simulink model "cruise_control_sdo"  (Simulink 8.0)
settings: Solver=FixedStepDiscrete  SolverMode=SingleTasking  StartTime=0.0  StopTime=50  FixedStep=0.01  RelTol=1e-3  AbsTol=1e-6
model workspace (MAT data in the model file):
  converter_data = [0  137.465208994  2.232; 0.1  137.065019157  2.075; 0.2  135.864449646  1.975; 0.3  135.664354728  1.846; 0.4  137.565256453  1.72; 0.5  140.366585312  1.564; 0.6  145.268910814  1.409; 0.7  152.872517717  1.254; 0.8  162.9773111  1.096; 0.81  164.27792807  1.08; 0.82  166.178829795  1.061; 0.83  167.979684062  1.043; 0.84  170.080680706  1.028; 0.85  172.781962105  1.012; 0.86  175.383196045  1.002; 0.87  179.585189333  1.002; 0.88  183.587087703  1.001; 0.89  189.890077635  0.998; 0.9  197.693779455  0.999; 0.92  215.902417037  1.001; 0.94  244.515990379  1.002]
  emap = [-40  -44  -49  -53  -57  -61  -65  -70  -74  -78  -82; 215  117  85  66  44  29  10  -2  -13  -22  -32; 245  208  178  148  122  104  85  66  48  33  18; 264  260  241  219  193  167  152  133  119  96  85; 264  279  282  275  260  238  223  208  189  171  152; 267  290  293  297  290  275  260  256  234  212  193; 267  297  305  305  305  301  293  282  267  249  226; 267  301  308  312  319  323  319  316  297  279  253; 267  301  312  319  327  327  327  327  312  293  267; 267  301  312  319  327  334  334  334  319  305  275]
  Iei = 0.0219914882836
  nevec = [800 1200 1600 2000 2400 2800 3200 3600 4000 4400 4800]
  p0 = 0.07934
  p1 = 0.07934
  thvec = [0; 20; 30; 40; 50; 60; 70; 80; 90; 100]
  vehicledata : num (value not decoded)
values from neighbouring files (symbols this model uses):
  cruise_ki = 0.01    [cruise_control_data.m]    (also in fxpdata_simulinkpackage.mat)
  cruise_kp = 0.02    [cruise_control_data.m]    (also in fxpdata_simulinkpackage.mat)
  target_max = 100    [cruise_control_data.m]    (also in fxpdata_simulinkpackage.mat)
  target_min = 30    [cruise_control_data.m]    (also in fxpdata_simulinkpackage.mat)
  throt_max = 100    [cruise_control_data.m]    (also in fxpdata_simulinkpackage.mat)
  throt_min = 0    [cruise_control_data.m]    (also in fxpdata_simulinkpackage.mat)
  vel_dec = 1    [cruise_control_data.m]    (also in fxpdata_simulinkpackage.mat)
  vel_inc = 1    [cruise_control_data.m]    (also in fxpdata_simulinkpackage.mat)
libraries: simulink x1
Description:
  | 幚憰梡僋儖?[僘僐儞僩???[儖儌僨儖
settings Model: MinMaxOverflowLogging=MinMaxAndOverflow  Creator=The MathWorks Inc.  LastModifiedBy=hualongy  CovMetricSettings=dcmtr  CovHTMLOptions=-aTS=1 -bRG=1 -bTC=1 -hTR=0 -nFC=0 -scm=1 -bcm=1 -xEv=0  ExtModeTrigMode=oneshot  ExtModeArmWhenConnect=off  ExtModeAutoUpdateStatusClock=off
settings DataIOCC: LimitDataPoints=off  SignalLoggingSaveFormat=ModelDataLogs  SaveOutput=off  SaveTime=off  SignalLoggingName=mysig
settings OptimizationCC: InlineParams=on  UseIntDivNetSlope=on  UseSpecifiedMinMax=on  InlineInvariantSignals=on  EnhancedBackFolding=on  PassReuseOutputArgsAs=Individual arguments  ZeroExternalMemoryAtStartup=off  ZeroInternalMemoryAtStartup=off  NoFixptDivByZeroProtection=on  EfficientFloat2IntCast=on  OptimizeModelRefInitCode=on  LifeSpan=1
settings DebuggingCC: SignalInfNanChecking=error  SaveWithParameterizedLinksMsg=none  CheckExecutionContextPreStartOutputMsg=on  CheckExecutionContextRuntimeOutputMsg=on  SolverPrmCheckMsg=none  SingleTaskRateTransMsg=error  IntegerOverflowMsg=error  FcnCallInpInsideContextMsg=EnableAllAsWarning  UniqueDataStoreMsg=error  BusObjectLabelMismatch=error  RootOutportRequireBusObject=error  AssertControl=DisableAll  StrictBusMsg=ErrorOnBusTreatedAsVector  BusNameAdapt=ErrorWithoutRepair  NonBusSignalsTreatedAsBus=error  LoggingUnavailableSignals=none
settings HardwareCC: ProdIntDivRoundTo=Zero  ProdEndianess=LittleEndian  ProdHWDeviceType=NEC->V850  TargetIntDivRoundTo=Zero  TargetEndianess=LittleEndian  TargetHWDeviceType=MATLAB Host
settings ModelReferenceCC: ModelReferenceNumInstancesAllowed=Single
settings SFSimCC: SFSimEcho=off  SimParseCustomCode=off
settings RTWCC: SystemTargetFile=ert.tlc  TemplateMakefile=ert_default_tmf  Description=Embedded Coder  GenerateReport=on  ProcessScript=ert_make_rtw_hook  IncludeHyperlinkInReport=on  LaunchReport=on  GenerateErtSFunction=on  CreateSILPILBlock=SIL  IncludeERTFirstTime=on  GenerateTraceInfo=on  GenerateTraceReport=on  GenerateTraceReportSl=on  GenerateTraceReportSf=on  GenerateTraceReportEml=on  RTWCompilerOptimization=On
settings CodeAppCC: IgnoreCustomStorageClasses=off  IgnoreTestpoints=on
settings ERTTargetCC: CodeReplacementLibrary=ANSI_C  UtilityFuncGeneration=Shared location  MultiwordLength=2048  GenerateSampleERTMain=on  IncludeMdlTerminateFcn=off  CombineSignalStateStructs=on  SuppressErrorStatus=on  SupportNonFinite=off  SupportComplex=off  PurelyIntegerCode=on  ParenthesesLevel=Maximum  InlinedParameterPlacement=NonHierarchical  ERTCustomFileTemplate=example_file_process.tlc  SuppressUnreachableDefaultCases=off
settings ConfigComp: Description=Design Verifier Custom Configuration Component  DVMaxProcessTime=3000  DVDisplayUnsatisfiableObjectives=on  DVMakeOutputFilesUnique=off  DVModelCoverageObjectives=MCDC  DVMaxTestCaseSteps=500  DVTestSuiteOptimization=CombinedObjectives (Nonlinear Extended)  DVSaveExpectedOutput=on  DVSaveHarnessModel=on  DVModelReferenceHarness=on  DVSaveReport=on

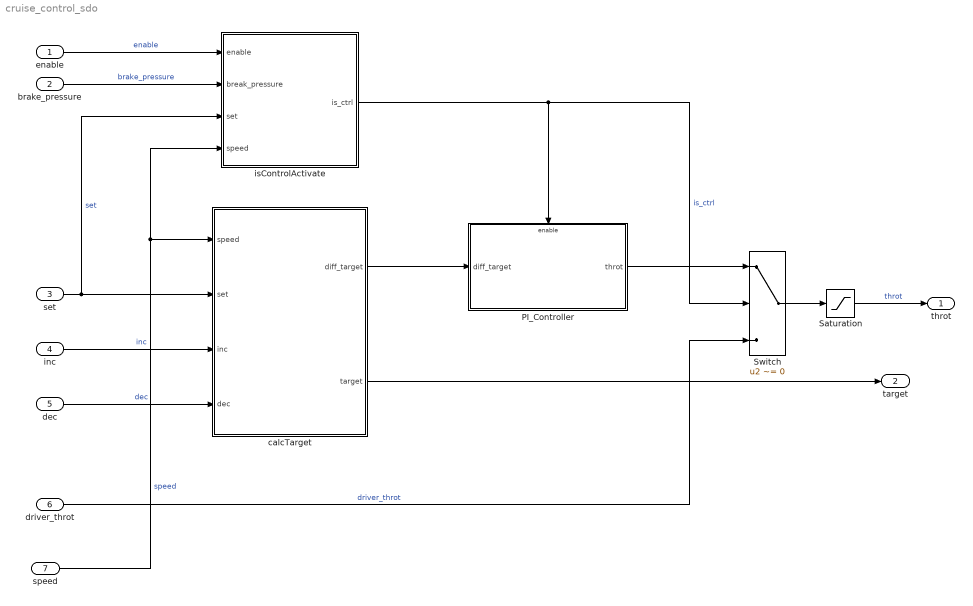
== system cruise_control_sdo ==
  enable : Inport  PortDimensions=1  Interpolate=off
  brake_pressure : Inport  Port=2  PortDimensions=1  Interpolate=off
  set : Inport  Port=3  PortDimensions=1  Interpolate=off
  inc : Inport  Port=4  PortDimensions=1  Interpolate=off
  dec : Inport  Port=5  PortDimensions=1  Interpolate=off
  driver_throt : Inport  Port=6  PortDimensions=1  Interpolate=off
  speed : Inport  Port=7  PortDimensions=1  Interpolate=off
  PI_Controller : Subsystem
  Saturation : Saturate  UpperLimit=throt_max  LowerLimit=throt_min  LinearizeAsGain=off  OutDataTypeStr=Inherit: Inherit via back propagation  RndMeth=Simplest
      settings: AttributesFormatString=<UpperLimit = %<UpperLimit>>\n<LowerLimit = %<LowerLimit>>
  Switch : Switch  Criteria=u2 ~= 0  OutDataTypeStr=Inherit: Inherit via back propagation
      settings: AttributesFormatString=<Criteria=%<Criteria>>
  calcTarget : Subsystem
  isControlActivate : Subsystem
  throt : Outport  PortDimensions=[1 1]
  target : Outport  Port=2  PortDimensions=[1 1]
  wires:
  isControlActivate/1(is_ctrl) -> Switch/2, PI_Controller/Enable  "is_ctrl"
  calcTarget/2(target) -> target/1
  calcTarget/1(diff_target) -> PI_Controller/1(diff_target)
  dec/1 -> calcTarget/4(dec)  "dec"
  speed/1 -> isControlActivate/4(speed), calcTarget/1(speed)  "speed"
  inc/1 -> calcTarget/3(inc)  "inc"
  set/1 -> isControlActivate/3(set), calcTarget/2(set)  "set"
  Switch/1 -> Saturation/1
  driver_throt/1 -> Switch/3  "driver_throt"
  brake_pressure/1 -> isControlActivate/2(break_pressure)  "brake_pressure"
  enable/1 -> isControlActivate/1(enable)  "enable"
  PI_Controller/1(throt) -> Switch/1
  Saturation/1 -> throt/1  "throt"

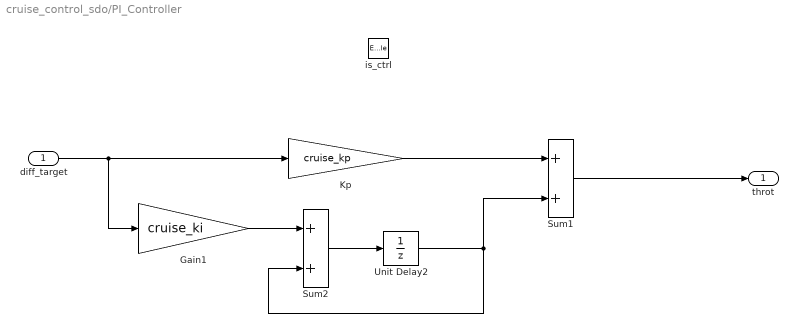
== system cruise_control_sdo/PI_Controller ==
  diff_target : Inport
  is_ctrl : EnablePort  StatesWhenEnabling=reset
  Gain1 : Gain  Gain=cruise_ki  OutDataTypeStr=Inherit: Same as input
  Kp : Gain  Gain=cruise_kp  ParamDataTypeStr=Inherit: Inherit from 'Gain'  OutDataTypeStr=Inherit: Inherit via back propagation
  Sum1 : Sum  OutDataTypeStr=Inherit: Inherit via back propagation
  Sum2 : Sum  OutDataTypeStr=Inherit: Inherit via back propagation
  Unit Delay2 : UnitDelay  SampleTime=-1
  throt : Outport
  wires:
  Unit Delay2/1 -> Sum2/2, Sum1/2
  Gain1/1 -> Sum2/1
  Kp/1 -> Sum1/1
  Sum1/1 -> throt/1
  diff_target/1 -> Gain1/1, Kp/1
  Sum2/1 -> Unit Delay2/1

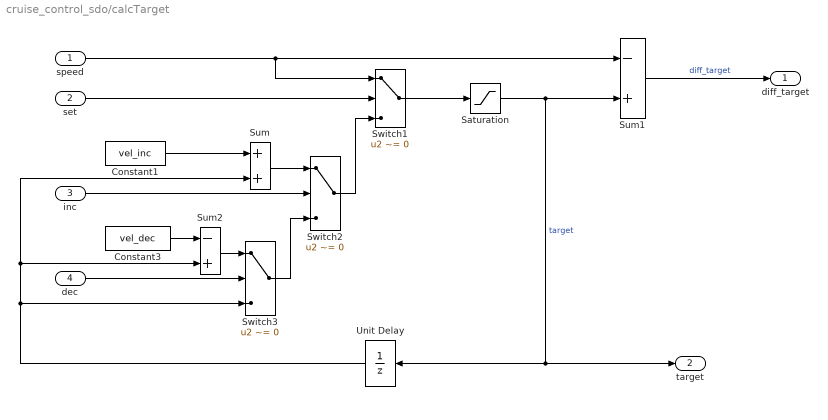
== system cruise_control_sdo/calcTarget ==
  speed : Inport
  set : Inport  Port=2
  inc : Inport  Port=3
  dec : Inport  Port=4
  Constant1 : Constant  Value=vel_inc  OutDataTypeStr=Inherit: Inherit via back propagation
  Constant3 : Constant  Value=vel_dec  OutDataTypeStr=Inherit: Inherit via back propagation
  Saturation : Saturate  UpperLimit=target_max  LowerLimit=target_min  LinearizeAsGain=off  RndMeth=Simplest
      settings: AttributesFormatString=<UpperLimit = %<UpperLimit>>\n<LowerLimit = %<LowerLimit>>
  Sum : Sum
  Sum1 : Sum  Inputs=-+  OutDataTypeStr=Inherit: Same as first input
  Sum2 : Sum  Inputs=-+
  Switch1 : Switch  Criteria=u2 ~= 0
      settings: AttributesFormatString=<Criteria=%<Criteria>>
  Switch2 : Switch  Criteria=u2 ~= 0
      settings: AttributesFormatString=<Criteria=%<Criteria>>
  Switch3 : Switch  Criteria=u2 ~= 0
      settings: AttributesFormatString=<Criteria=%<Criteria>>
  Unit Delay : UnitDelay  SampleTime=-1
  diff_target : Outport
  target : Outport  Port=2
  wires:
  Saturation/1 -> Sum1/2, target/1, Unit Delay/1  "target"
  set/1 -> Switch1/2
  speed/1 -> Switch1/1, Sum1/1
  inc/1 -> Switch2/2
  Constant1/1 -> Sum/1
  Sum/1 -> Switch2/1
  dec/1 -> Switch3/2
  Constant3/1 -> Sum2/1
  Sum2/1 -> Switch3/1
  Switch2/1 -> Switch1/3
  Switch3/1 -> Switch2/3
  Unit Delay/1 -> Switch3/3, Sum2/2, Sum/2
  Switch1/1 -> Saturation/1
  Sum1/1 -> diff_target/1  "diff_target"

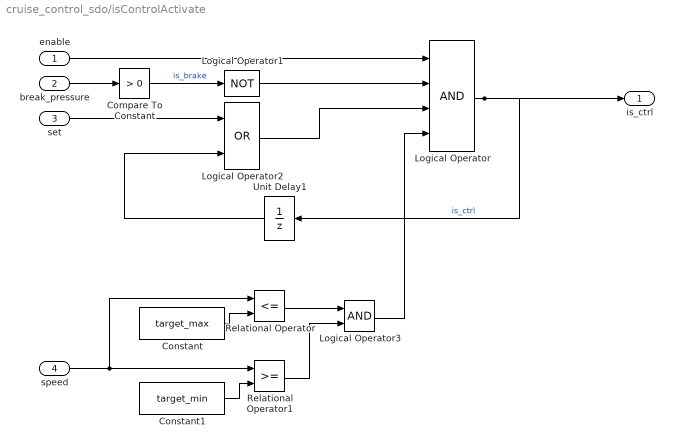
== system cruise_control_sdo/isControlActivate ==
  enable : Inport
  break_pressure : Inport  Port=2
  set : Inport  Port=3
  speed : Inport  Port=4
  Compare To Constant : simulink/Logic and Bit Operations/Compare To Constant  relop=>  const=0  OutDataTypeStr=uint8
  Constant : Constant  Value=target_max
  Constant1 : Constant  Value=target_min
  Logical Operator : Logic  Inputs=4  AllPortsSameDT=off  OutDataTypeStr=boolean
  Logical Operator1 : Logic  Operator=NOT  AllPortsSameDT=off  OutDataTypeStr=boolean
  Logical Operator2 : Logic  Operator=OR  AllPortsSameDT=off  OutDataTypeStr=boolean
  Logical Operator3 : Logic  AllPortsSameDT=off  OutDataTypeStr=boolean
  Relational Operator : RelationalOperator  Operator=<=  OutDataTypeStr=boolean
  Relational Operator1 : RelationalOperator  OutDataTypeStr=boolean
  Unit Delay1 : UnitDelay  SampleTime=-1
  is_ctrl : Outport
  wires:
  Compare To Constant/1 -> Logical Operator1/1  "is_brake"
  Constant/1 -> Relational Operator/2
  Logical Operator3/1 -> Logical Operator/4
  Relational Operator1/1 -> Logical Operator3/2
  Relational Operator/1 -> Logical Operator3/1
  speed/1 -> Relational Operator/1, Relational Operator1/1
  Constant1/1 -> Relational Operator1/2
  break_pressure/1 -> Compare To Constant/1
  enable/1 -> Logical Operator/1
  set/1 -> Logical Operator2/1
  Logical Operator1/1 -> Logical Operator/2
  Logical Operator2/1 -> Logical Operator/3
  Unit Delay1/1 -> Logical Operator2/2
  Logical Operator/1 -> is_ctrl/1, Unit Delay1/1  "is_ctrl"
